simulink model "Task5_servo_controller"  (R2023b)
settings: Solver=VariableStepAuto  StartTime=0.0  StopTime=25  RelTol=1e-3
values from neighbouring files (symbols this model uses):
  A = [-1.7  -0.25  0; 23  -30  20; 0  -250  -720]    [A.mat]
  B = [3  0; -103  0; 0  -790]    [B.mat]
  C = [0  1  0; 0  0  1]    [C.mat]
  K1 = K(:,1:3)    [Task5_servo_control.m]    (also in Task6_servo_control.m)
  K2 = K(:,4:5)    [Task5_servo_control.m]    (also in Task6_servo_control.m)
  L = L_bar*T    [Task3_LQR_observer.m]    (also in Task5_servo_control.m)
settings Model: Creator=25039  LastModifiedBy=25039

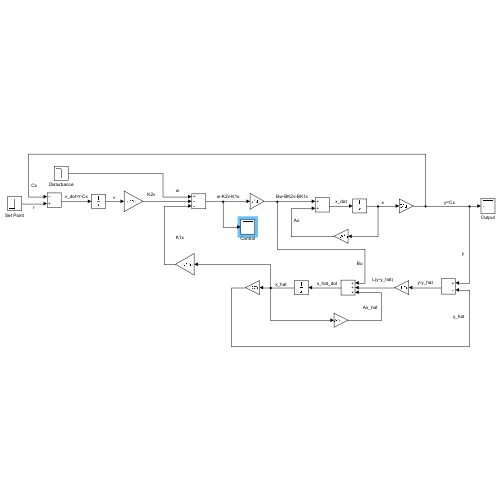
[thumbnail: Simulink's stored preview of the top-level diagram]
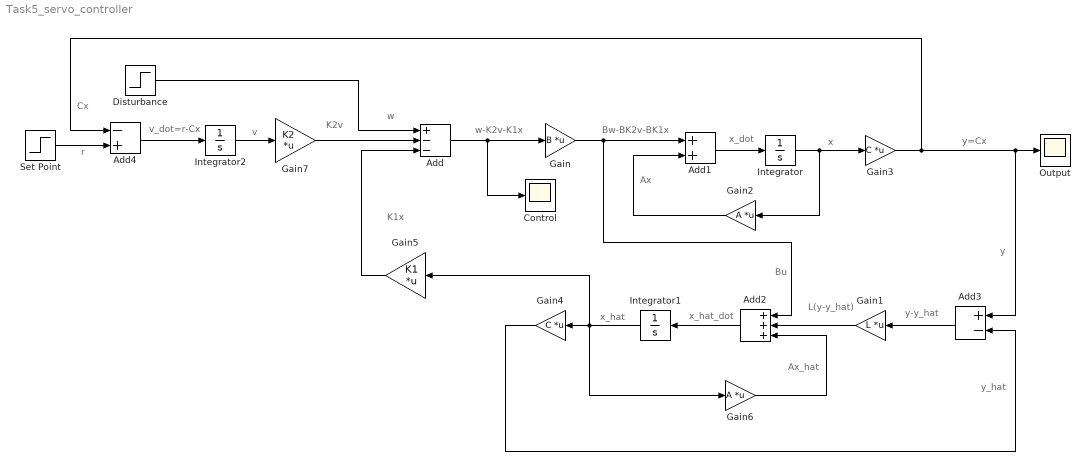
== system Task5_servo_controller ==
  note: K2v
  note: K1x
  note: v
  note: v_dot=r-Cx
  note: Cx
  note: w
  note: y-y_hat
  note: L(y-y_hat)
  note: x_hat
  note: x_hat_dot
  note: y_hat
  note: y
  note: y=Cx
  note: x
  note: x_dot
  note: Ax
  note: Bw-BK2v-BK1x
  note: w-K2v-K1x
  note: r
  note: Bu
  note: Ax_hat
  Add : Sum  Inputs=+--
  Add1 : Sum
  Add2 : Sum  Inputs=+++
  Add3 : Sum  Inputs=+-
  Add4 : Sum  Inputs=-+
  Control : Scope
  Disturbance : Step  Time=10  Before=[0, 0]  After=[-2, 5]
  Gain : Gain  Gain=B  Multiplication=Matrix(K*u)
  Gain1 : Gain  Gain=L  Multiplication=Matrix(K*u)
  Gain2 : Gain  Gain=A  Multiplication=Matrix(K*u)
  Gain3 : Gain  Gain=C  Multiplication=Matrix(K*u)
  Gain4 : Gain  Gain=C  Multiplication=Matrix(K*u)
  Gain5 : Gain  Gain=K1  Multiplication=Matrix(K*u)
  Gain6 : Gain  Gain=A  Multiplication=Matrix(K*u)
  Gain7 : Gain  Gain=K2  Multiplication=Matrix(K*u)
  Integrator : Integrator  InitialCondition=[1,100,200]
  Integrator1 : Integrator
  Integrator2 : Integrator
  Output : Scope
  Set Point : Step  Time=0  Before=[0, 0]  After=[100, 150]
  wires:
  Add/1 -> Control/1, Gain/1
  Gain/1 -> Add2/1, Add1/1
  Add1/1 -> Integrator/1
  Gain3/1 -> Add4/1, Add3/1, Output/1
  Integrator/1 -> Gain2/1, Gain3/1
  Gain2/1 -> Add1/2
  Add3/1 -> Gain1/1
  Gain1/1 -> Add2/2
  Add2/1 -> Integrator1/1
  Integrator1/1 -> Gain6/1, Gain5/1, Gain4/1
  Gain5/1 -> Add/3
  Gain4/1 -> Add3/2
  Gain6/1 -> Add2/3
  Disturbance/1 -> Add/1
  Set Point/1 -> Add4/2
  Add4/1 -> Integrator2/1
  Gain7/1 -> Add/2
  Integrator2/1 -> Gain7/1
